simulink model "Debugging_Quadcopter"  (R2019b)
settings: Solver=VariableStepAuto  StartTime=0.0  StopTime=10.0  RelTol=1e-3
settings Model: Creator=7385281  LastModifiedBy=7385281

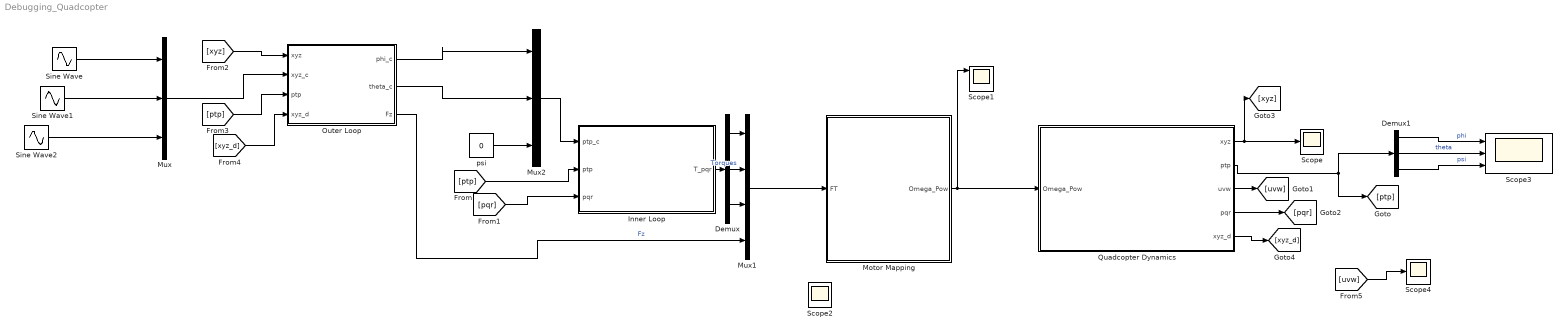
== system Debugging_Quadcopter ==
  Demux : Demux  Outputs=3
  Demux1 : Demux  Outputs=3
  Inner Loop : Subsystem
  Motor Mapping : MATLAB Function  TreatAsAtomicUnit=on
  Mux : Mux  Inputs=3
  Mux1 : Mux
  Mux2 : Mux  Inputs=3
  Outer Loop : Subsystem
  Quadcopter Dynamics : Subsystem
  Scope : Scope
  Scope1 : Scope  NumInputPorts=3
  Scope2 : Scope
  Scope3 : Scope  NumInputPorts=3
  Scope4 : Scope
  Sine Wave : Sin  SampleTime=0
  Sine Wave1 : Sin  SampleTime=0
  Sine Wave2 : Sin  SampleTime=0
  psi : Constant  Value=0
  wires:
  Sine Wave/1 -> Mux/1
  Sine Wave1/1 -> Mux/2
  Sine Wave2/1 -> Mux/3
  Quadcopter Dynamics/1(xyz) -> [xyz], Scope/1
  Quadcopter Dynamics/3(uvw) -> [uvw]
  Demux/3 -> Mux1/3
  Demux/2 -> Mux1/2
  Demux/1 -> Mux1/1
  Outer Loop/3(Fz) -> Mux1/4  "Fz"
  Inner Loop/1(T_pqr) -> Demux/1  "Torques"
  Quadcopter Dynamics/2(ptp) -> Demux1/1, [ptp]
  Demux1/1 -> Scope3/1  "phi"
  Demux1/2 -> Scope3/2  "theta"
  Demux1/3 -> Scope3/3  "psi"
  Quadcopter Dynamics/4(pqr) -> [pqr]
  [ptp] -> Inner Loop/2(ptp)
  [pqr] -> Inner Loop/3(pqr)
  Motor Mapping/1(Omega_Pow) -> Quadcopter Dynamics/1(Omega_Pow), Scope1/1
  Mux/1 -> Outer Loop/2(xyz_c)
  [xyz] -> Outer Loop/1(xyz)
  [ptp] -> Outer Loop/3(ptp)
  Outer Loop/1(phi_c) -> Mux2/1
  Outer Loop/2(theta_c) -> Mux2/2
  Mux2/1 -> Inner Loop/1(ptp_c)
  psi/1 -> Mux2/3
  Quadcopter Dynamics/5(xyz_d) -> [xyz_d]
  [xyz_d] -> Outer Loop/4(xyz_d)
  [uvw] -> Scope4/1
  Mux1/1 -> Motor Mapping/1(FT)

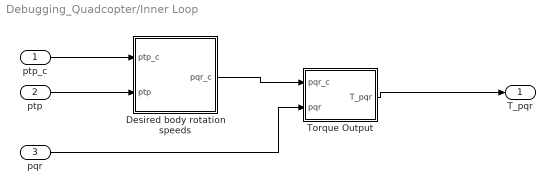
== system Debugging_Quadcopter/Inner Loop ==
  ptp_c : Inport
  ptp : Inport  Port=2
  pqr : Inport  Port=3
  Desired body rotation speeds : MATLAB Function  TreatAsAtomicUnit=on
  Torque Output : MATLAB Function  TreatAsAtomicUnit=on
  T_pqr : Outport
  wires:
  ptp/1 -> Desired body rotation speeds/2(ptp)
  pqr/1 -> Torque Output/2(pqr)
  Torque Output/1(T_pqr) -> T_pqr/1
  ptp_c/1 -> Desired body rotation speeds/1(ptp_c)
  Desired body rotation speeds/1(pqr_c) -> Torque Output/1(pqr_c)

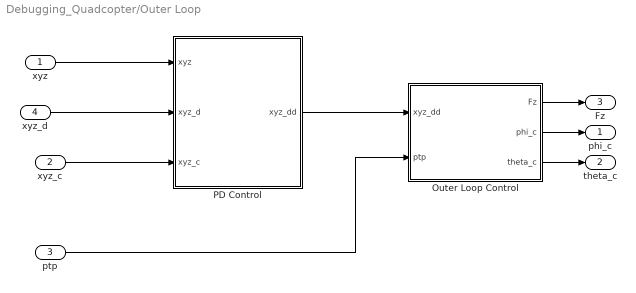
== system Debugging_Quadcopter/Outer Loop ==
  xyz : Inport
  xyz_c : Inport  Port=2
  ptp : Inport  Port=3
  xyz_d : Inport  Port=4
  Outer Loop Control : MATLAB Function  TreatAsAtomicUnit=on
  PD Control : MATLAB Function  TreatAsAtomicUnit=on
  phi_c : Outport
  theta_c : Outport  Port=2
  Fz : Outport  Port=3
  wires:
  PD Control/1(xyz_dd) -> Outer Loop Control/1(xyz_dd)
  xyz/1 -> PD Control/1(xyz)
  xyz_c/1 -> PD Control/3(xyz_c)
  ptp/1 -> Outer Loop Control/2(ptp)
  Outer Loop Control/1(Fz) -> Fz/1
  Outer Loop Control/2(phi_c) -> phi_c/1
  Outer Loop Control/3(theta_c) -> theta_c/1
  xyz_d/1 -> PD Control/2(xyz_d)

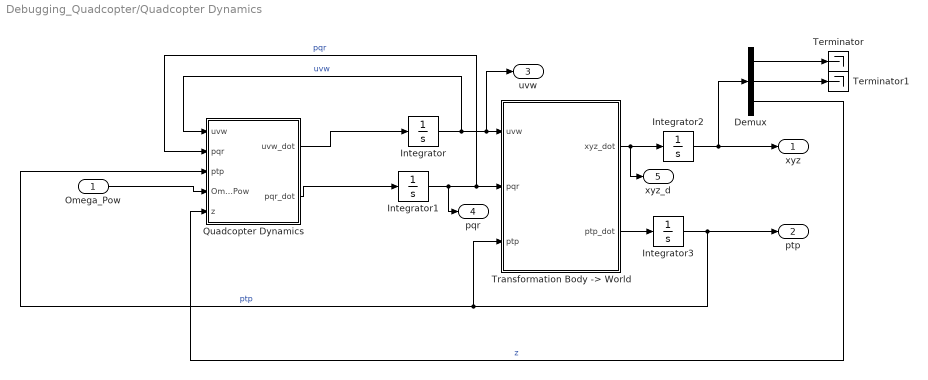
== system Debugging_Quadcopter/Quadcopter Dynamics ==
  Omega_Pow : Inport
  Demux : Demux  Outputs=3
  Integrator : Integrator  InitialCondition=[0.001; 0.001; 0.001]
  Integrator1 : Integrator  InitialCondition=[0.001;0.001;0.001]
  Integrator2 : Integrator
  Integrator3 : Integrator  InitialCondition=[0.001; 0.001; 0.001]
  Quadcopter Dynamics : MATLAB Function  TreatAsAtomicUnit=on
  Terminator : Terminator
  Terminator1 : Terminator
  "Transformation Body -> World" : MATLAB Function  TreatAsAtomicUnit=on
  xyz : Outport
  ptp : Outport  Port=2
  uvw : Outport  Port=3
  pqr : Outport  Port=4
  xyz_d : Outport  Port=5
  wires:
  "Transformation Body -> World"/1(xyz_dot) -> xyz_d/1, Integrator2/1
  Quadcopter Dynamics/2(pqr_dot) -> Integrator1/1
  Integrator3/1 -> ptp/1, "Transformation Body -> World"/3(ptp), Quadcopter Dynamics/3(ptp)  "ptp"
  "Transformation Body -> World"/2(ptp_dot) -> Integrator3/1
  Omega_Pow/1 -> Quadcopter Dynamics/4(Omega_Pow)
  Quadcopter Dynamics/1(uvw_dot) -> Integrator/1
  Integrator1/1 -> pqr/1, Quadcopter Dynamics/2(pqr), "Transformation Body -> World"/2(pqr)  "pqr"
  Integrator/1 -> Quadcopter Dynamics/1(uvw), uvw/1, "Transformation Body -> World"/1(uvw)  "uvw"
  Integrator2/1 -> Demux/1, xyz/1
  Demux/3 -> Quadcopter Dynamics/5(z)  "z"
  Demux/1 -> Terminator/1
  Demux/2 -> Terminator1/1

== matlab function Debugging_Quadcopter/Quadcopter Dynamics/Transformation Body -> World ==
  data: uvw input; xyz_dot output; pqr input; ptp_dot output; ptp input
function [xyz_dot,ptp_dot] = fcn(uvw,pqr,ptp)
%{
This code transforms the body frame velocities to the world frame
velocities

INPUTS:
    uvw - 3x1 vector of body transl. velocities u, v, w
    pqr - 3x1 vector of body rotat. velocities, p, q, r

OUTPUTS:
    xyz_dot - 3x1 vector of world transl. velocities x_dot, y_dot, z_dot
    ptp_dot -3x1 vector of world derivative orientations, phi, theta, psi

%}
% CONSTANTS
m = 2.3;              % Mass [kg]
L = 0.7;              % Lever arm length [m]
Ixx = 8.04*10^(-3);   % Body inertia of x axis [kg*m^2]
Iyy = 8.46*10^(-3);   % Body inertia of y axis [kg*m^2]
Izz = 14.68*10^(-3);  % Body inertia of y axis [kg*m^2]
k_f = 0.65016*10^(-3);    % Force Coeffecient [N/(rad/s)^2]
k_t = 0.82218*10^(-5);     % Torque Coeffecient [N/(rad/s)^2]
k1 = 20;              % Motor model coeffecient
k2 = 0.01;            % Motor model coeffecient
k3 = 3.5;             % Motor model coeffecient
z_i = 0.003;          % Elastic deformation [m]
k_i = 6000;           % Elastic Coeffecient of gear [N/m]

% INITIALIZATION
phi = ptp(1);
theta = ptp(2);
psi = ptp(3);

% MAIN CODE

% Positional transformation
xyz_dot = [cos(theta)*cos(psi) -cos(phi)*sin(psi)+sin(phi)*sin(theta)*cos(psi) sin(phi)*sin(psi)+cos(phi)*sin(theta)*cos(psi);...
    cos(theta)*sin(psi) cos(phi)*cos(psi)+sin(phi)*sin(theta)*sin(psi) -sin(phi)*cos(psi)+cos(phi)*sin(theta)*sin(psi);...
    -sin(theta) sin(phi)*cos(theta) cos(phi)*cos(theta)]*uvw;


% Orientation transformation
ptp_dot = [1 sin(phi)*tan(theta) cos(phi)*tan(theta); 0 cos(phi) -sin(phi); 0 sin(phi)/cos(theta) cos(phi)/cos(theta)]*pqr;

== matlab function Debugging_Quadcopter/Quadcopter Dynamics/Quadcopter Dynamics ==
  data: uvw input; uvw_dot output; pqr input; ptp input; pqr_dot output; Omega_Pow input; z input
function [uvw_dot, pqr_dot] = fcn(uvw,pqr,ptp,Omega_Pow,z)
%{
This code simulates the body dyanics of a quadcopter
INPUTS:
    uvw - 3x1 vector of body fixed translation velocities u, v, w
    pqr - 3x1 vector of body fixed rotation velocities p, q, r
    ptp - 3x1 vector of world fixed orientations phi, theta, psi
    Omega_Pow - 4x1 vector of  propeller angular velocities

OUTPUTS:
    uvw_dot - 3x1 vector of derivatives of body velocities u, v, w
    pqr_dot - 3x1 vector of derivatives of body rotation velocities, p, q, r
%}

% CONSTANTS
m = 2.3;              % Mass [kg]
g = 9.81;             % Gravity [m/s^2]
L = 0.7;              % Lever arm length [m]
Ixx = 8.04*10^(-3);   % Body inertia of x axis [kg*m^2]
Iyy = 8.46*10^(-3);   % Body inertia of y axis [kg*m^2]
Izz = 14.68*10^(-3);  % Body inertia of y axis [kg*m^2]
k_f = 0.65016*10^(-3);    % Force Coeffecient [N/(rad/s)^2]
k_t = 0.82218*10^(-5);     % Torque Coeffecient [N/(rad/s)^2]
k1 = 20;              % Motor model coeffecient
k2 = 0.01;            % Motor model coeffecient
k3 = 3.5;             % Motor model coeffecient
z_i = 0.003;          % Elastic deformation [m]
k_i = 6000;           % Elastic Coeffecient of gear [N/m]

% INITIALIZATION

% Gets values from matrix
u = uvw(1);
v = uvw(2);
w = uvw(3);

p = pqr(1);
q = pqr(2);
r = pqr(3);

phi = ptp(1);
theta = ptp(2);
psi = ptp(3);

% Deformation of landing gear
% If on the ground/landing
if (z_i - z)> 0
    delta = 1;
% If in the air
else
    delta = 0;
end




% MAIN CODE

% Uses angular speeds of propellers to map forces
FT = [-L*k_f L*k_f L*k_f -L*k_f;...
    -L*k_f L*k_f -L*k_f L*k_f;...
    k_t k_t -k_t -k_t;...
    k_f k_f k_f k_f]*Omega_Pow;

% Sets forces
Tp = FT(1);
Tq = FT(2);
Tr = FT(3);
Fz = FT(4);

% Body Fixed Translational Dynamics
uvw_dot = [-r*v+q*w; r*u-p*w; -q*u+p*v]+[0; 0; Fz/m]+[g*sin(theta); -g*cos(theta)*sin(psi); -g*cos(theta)*sin(psi)]+[0; 0; k_i*(z_i-z)*delta];

% Body Fixed Rotational Dynamics
pqr_dot = -[q*r*(Izz-Iyy)/Ixx; p*r*(Ixx-Izz)/Iyy; p*q*(Iyy-Ixx)/Izz]+[Tp/Ixx; Tq/Iyy; Tr/Izz];

== matlab function Debugging_Quadcopter/Motor Mapping ==
  data: FT input; Omega_Pow output
function Omega_Pow = fcn(FT)
%{
This function takes the desired forces and maps them to the proppeller
speed. This is important because angular velocity is easily measured
compared to the thrust forces

INPUTS:
    FT - 4x1 desired force vector Tp, Tq, Tr, Fz

OUTPUTS:
    Omega_Pow2 = 4x1 vector of  angular velocities of propellers
%}
% CONSTANTS
m = 2.3;              % Mass [kg]
L = 0.7;              % Lever arm length [m]
Ixx = 8.04*10^(-3);   % Body inertia of x axis [kg*m^2]
Iyy = 8.46*10^(-3);   % Body inertia of y axis [kg*m^2]
Izz = 14.68*10^(-3);  % Body inertia of y axis [kg*m^2]
k_f = 0.65016*10^(-3);    % Force Coeffecient [N/(rad/s)^2]
k_t = 0.82218*10^(-5);     % Torque Coeffecient [N/(rad/s)^2]
k1 = 20;              % Motor model coeffecient
k2 = 0.01;            % Motor model coeffecient
k3 = 3.5;             % Motor model coeffecient
z_i = 0.003;          % Elastic deformation [m]
k_i = 6000;           % Elastic Coeffecient of gear [N/m]

% INITIALIZATION
Tp = FT(1);
Tq = FT(2);
Tr = FT(3);
Fz = FT(4);

% MAIN CODE

% Calculates Omega_Pow
Omega_Pow =[-0.25 -0.25 0.25 0.25;...
    0.25 0.25 0.25 0.25;...
    0.25 -0.25 -0.25 0.25;...
    -0.25 0.25 -0.25 0.25]*[Tp/(L*k_f); Tq/(L*k_f); Tr/(L*k_t); Fz/k_f];

== matlab function Debugging_Quadcopter/Inner Loop/Desired body rotation speeds ==
  data: ptp_c input; pqr_c output; ptp input
function pqr_c = fcn(ptp_c,ptp)
%{
This function takes in the desired attidue angles and the attitude angles
of the quadcopter and determines the desired body rotation velocities
% INPUTS:
    ptp_c - 3x1 vector of desired attitude (orientation) angles
    ptp - 3x1 vector of attitude angle phi, theta, psi
% OUTPUTS 
    pqr_c - 3x1 vector of desired body frame rotation velocities p, q, r
%}
% CONSTANTS:
m = 2.3;              % Mass [kg]
L = 0.7;              % Lever arm length [m]
Ixx = 8.04*10^(-3);   % Body inertia of x axis [kg*m^2]
Iyy = 8.46*10^(-3);   % Body inertia of y axis [kg*m^2]
Izz = 14.68*10^(-3);  % Body inertia of y axis [kg*m^2]
k_f = 0.65016*10^(-3);    % Force Coeffecient [N/(rad/s)^2]
k_t = 0.82218*10^(-5);     % Torque Coeffecient [N/(rad/s)^2]
k1 = 20;              % Motor model coeffecient
k2 = 0.01;            % Motor model coeffecient
k3 = 3.5;             % Motor model coeffecient
z_i = 0.003;          % Elastic deformation [m]
k_i = 6000;           % Elastic Coeffecient of gear [N/m]

% INITIALIZATION
phi = ptp(1);
theta = ptp(2);
psi = ptp(3);

phi_c = ptp_c(1);
theta_c = ptp_c(2);
psi_c = ptp_c(3);

% CONTROL CONSTANTS
nat_freq = 10;   % Natural Frequency [Hz]
nat_freq = nat_freq*6.28;   % [rad/s]

damp = 0.7;    % Damping Ratio

k_phi = nat_freq/(2*damp);
k_theta = k_phi;
k_psi = k_phi;

% MAIN CODE

% Desired body frame rotation velocities
pqr_c = inv([1 sin(psi)*tan(theta) cos(psi)*tan(theta);...
    0 cos(psi) -sin(psi);...
    0 sin(psi)/cos(theta) cos(psi)/cos(theta)])...
    *[k_psi*(phi_c-psi);...
    k_theta*(theta_c-theta);...
    k_psi*(psi_c-psi)];

== matlab function Debugging_Quadcopter/Inner Loop/Torque Output ==
  data: pqr_c input; T_pqr output; pqr input
function T_pqr = fcn( pqr_c,pqr)

% CONSTANTS:
m = 2.3;              % Mass [kg]
L = 0.7;              % Lever arm length [m]
Ixx = 8.04*10^(-3);   % Body inertia of x axis [kg*m^2]
Iyy = 8.46*10^(-3);   % Body inertia of y axis [kg*m^2]
Izz = 14.68*10^(-3);  % Body inertia of y axis [kg*m^2]
k_f = 0.65016*10^(-3);    % Force Coeffecient [N/(rad/s)^2]
k_t = 0.82218*10^(-5);     % Torque Coeffecient [N/(rad/s)^2]
k1 = 20;              % Motor model coeffecient
k2 = 0.01;            % Motor model coeffecient
k3 = 3.5;             % Motor model coeffecient
z_i = 0.003;          % Elastic deformation [m]
k_i = 6000;           % Elastic Coeffecient of gear [N/m]

% CONTROL CONSTANTS
nat_freq = 10;   % Natural Frequency [Hz]
nat_freq = nat_freq*6.28;   % [rad/s]

damp = 0.7;    % Damping Ratio

k_p = 2*nat_freq*damp;
k_q = k_p;

nat_freq2 = 2;  % Natural Frequency of yaw attidude
k_r = 2*nat_freq2*damp;


% INITIALIZATION
p_c = pqr_c(1);
q_c = pqr_c(2);
r_c = pqr_c(3);

p = pqr(1);
q = pqr(2);
r = pqr(3);

% MAIN CODE

T_pqr = [k_p*(p_c-p)*Ixx; k_q*(q_c-q)*Iyy; k_r*(r_c-r)*Izz];

== matlab function Debugging_Quadcopter/Outer Loop/Outer Loop Control ==
  data: xyz_dd input; Fz output; ptp input; phi_c output; theta_c output
function [Fz, phi_c, theta_c] = fcn(xyz_dd,ptp)
%{
This function takes the control inputs xyz_dd and the oreintation of the
quadcopter to determine the Fz and phi and theta control
inputs

% INPUTS:
    xyz_dd - 3x1 vector of control input accelerations
    ptp - 3x1 vector of world frame orientation

% OUTPUTS:
    Fz - desired force in Z
    phi_c - desired orientation in phi
    theta_c - desired orientation in theta
%}
% CONSTANTS
m = 2.3;              % Mass [kg]
g = 9.81;             % Gravity [m/s^2]
L = 0.7;              % Lever arm length [m]
Ixx = 8.04*10^(-3);   % Body inertia of x axis [kg*m^2]
Iyy = 8.46*10^(-3);   % Body inertia of y axis [kg*m^2]
Izz = 14.68*10^(-3);  % Body inertia of y axis [kg*m^2]
k_f = 0.65016*10^(-3);    % Force Coeffecient [N/(rad/s)^2]
k_t = 0.82218*10^(-5);     % Torque Coeffecient [N/(rad/s)^2]
k1 = 20;              % Motor model coeffecient
k2 = 0.01;            % Motor model coeffecient
k3 = 3.5;             % Motor model coeffecient
z_i = 0.003;          % Elastic deformation [m]
k_i = 6000;           % Elastic Coeffecient of gear [N/m]

% INITIALIZATION
x_dd = xyz_dd(1);
y_dd = xyz_dd(2);
z_dd = xyz_dd(3);

phi = ptp(1);
theta = ptp(2);
psi = ptp(3);

% Calculates Desired Force in Z
Fz = (z_dd+g)/m;

% Calculates desired phi angle
phi_c = (x_dd*sin(psi)-y_dd*cos(psi))*m/Fz;

% Calculates desired theta angle
theta_c = (x_dd*cos(psi)-y_dd*sin(psi))*m/Fz;

== matlab function Debugging_Quadcopter/Outer Loop/PD Control ==
  data: xyz input; xyz_dd output; xyz_d input; xyz_c input
function xyz_dd = fcn(xyz,xyz_d,xyz_c)
%{
This function uses PD control to determine control vector of accelereations

INPUTS:
    xyz - 3x1 vector of quadcopter position
    xyz_c - 3x1 vector of desired quadcopter position
    xyz_dd - 3x1 vector of quadcopter world velocities

OUTPUTS:
    xyz_dd - 3x1 vector of control accelerations
%}
% CONTROL CONSTANTS:
nat_freq = 1;   % Natural Frequency [Hz]
nat_freq = nat_freq*6.28;   % [rad/s]

damp = 0.72;    % Damping Ratio

k_x = nat_freq/(2*damp);
k_y = k_x;
k_z = k_x;

k_u = 2*nat_freq*damp;
k_v = k_u;
k_w = k_u;

% INITIALIZATION
x = xyz(1);
y = xyz(2);
z = xyz(3);

x_c = xyz_c(1);
y_c = xyz_c(2);
z_c = xyz_c(3);

% MAIN CODE

% Calculates control vector acceleration
xyz_dd = [-k_u; -k_v; -k_w].*xyz_d-[k_u; k_v; k_w].*[k_x; k_y; k_z].*[x-y_c; y-y_c; z-z_c];
